simulink model "P41"  (R2015b)
settings: Solver=VariableStepAuto  StartTime=0.0  StopTime=10  RelTol=1e-3
libraries: fl_lib x19, nesl_utility x3
settings Model: Creator=xmax1946  LastModifiedBy=xmax1946

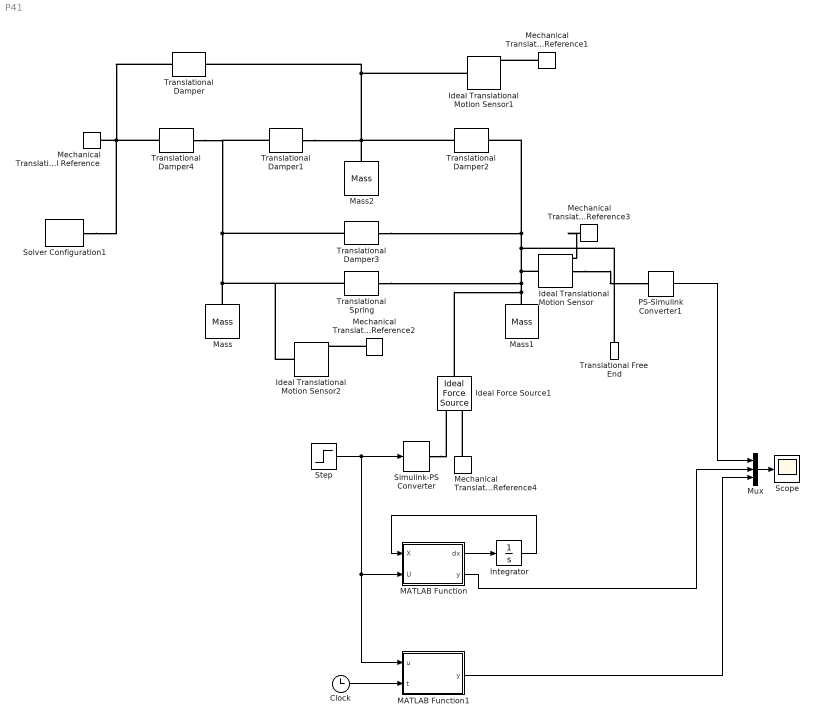
== system P41 ==
  Clock : Clock
  Ideal Force Source1 : fl_lib/Mechanical/Mechanical Sources/Ideal Force Source
  Ideal Translational Motion Sensor : fl_lib/Mechanical/Mechanical Sensors/Ideal Translational Motion Sensor  offset=0 m
  Ideal Translational Motion Sensor1 : fl_lib/Mechanical/Mechanical Sensors/Ideal Translational Motion Sensor  offset=0 m
  Ideal Translational Motion Sensor2 : fl_lib/Mechanical/Mechanical Sensors/Ideal Translational Motion Sensor  offset=0 m
  Integrator : Integrator  InitialCondition=[0;0;0;0;0;0]
  MATLAB Function : MATLAB Function  TreatAsAtomicUnit=on
  MATLAB Function1 : MATLAB Function  TreatAsAtomicUnit=on
  Mass : fl_lib/Mechanical/Translational Elements/Mass  mass=2 kg  v_specify=off  v_priority=None  v=0 m/s  f_specify=off  f_priority=None  f=0 N
  Mass1 : fl_lib/Mechanical/Translational Elements/Mass  mass=1 kg  v_specify=off  v_priority=None  v=0 m/s  f_specify=off  f_priority=None  f=0 N
  Mass2 : fl_lib/Mechanical/Translational Elements/Mass  mass=1 kg  v_specify=off  v_priority=None  v=0 m/s  f_specify=off  f_priority=None  f=0 N
  Mechanical Translational Reference{,1..4} (5 alike) : fl_lib/Mechanical/Translational Elements/Mechanical Translational Reference
  Mux : Mux  Inputs=3
  PS-Simulink Converter1 : nesl_utility/PS-Simulink Converter  PhysicalDomain=network_engine_domain  SubClassName=ps_output  LeftPortType=input  RightPortType=output  PseudoPeriodic=off  Frequencies=[]  Unit=1  AffineConversion=off
  Scope : Scope
  Simulink-PS Converter : nesl_utility/Simulink-PS Converter  PhysicalDomain=network_engine_domain  SubClassName=ps_input  LeftPortType=input  RightPortType=output  PseudoPeriodic=off  Frequencies=[]  NoiseDistribution=none  NoiseParameters=[]  Unit=1  AffineConversion=off  InputFiltering=off  SimscapeFilterOrder=1  InputFilterTimeConstant=0.001  UdotUserProvided=1
  Solver Configuration1 : nesl_utility/Solver Configuration  PhysicalDomain=network_engine_domain  SubClassName=solver  LeftPortType=input  RightPortType=generic  Accelerate=off  Tones=[]  Harmonics=[]  SimulateNoise=off  Profile=off  UseLocalSampling=off  EnableSwitchedLinearOptims=on  FrequencyDomain=off  UseCCode=off  RelTol=0.001  AbsTol=1e-06  MinStep=1e-09  ToWorkspace=off  RevertToSquareIcSolve=off  NumHomotopyIterations=100  PhasorMode=off  PhasorModeNumHarmonics=1  DoDC=off  ResidualTolerance=1e-09  UseLocalSolver=off  LocalSolverChoice=NE_BACKWARD_EULER_ADVANCER  LocalSolverSampleTime=0.001  DoFixedCost=off  MaxNonlinIter=3  MaxModeIter=2  LinearAlgebra=Sparse  DelaysMemoryBudget=1024  AutomaticFiltering=on  FilteringTimeConstant=0.001
  Step : Step  SampleTime=0
  Translational Damper{,1..4} (5 alike) : fl_lib/Mechanical/Translational Elements/Translational Damper  D=1 N/(m/s)  v_specify=off  v_priority=None  v=0 m/s  f_specify=off  f_priority=None  f=0 N
  Translational Free End : fl_lib/Mechanical/Translational Elements/Translational Free End  v_specify=off  v_priority=None  v=0 m/s
  Translational Spring : fl_lib/Mechanical/Translational Elements/Translational Spring  spr_rate=2 N/m  v_specify=off  v_priority=None  v=0 m/s  f_specify=off  f_priority=None  f=0 N  x_specify=off  x_priority=None  x=0 m
  wires:
  Step/1 -> MATLAB Function1/1(u), MATLAB Function/2(U), Simulink-PS Converter/1
  MATLAB Function/1(dx) -> Integrator/1
  MATLAB Function/2(y) -> Mux/2
  PS-Simulink Converter1/1 -> Mux/1
  Mux/1 -> Scope/1
  Integrator/1 -> MATLAB Function/1(X)
  MATLAB Function1/1(y) -> Mux/3
  Clock/1 -> MATLAB Function1/2(t)
  connections:
  Translational Damper4/LConn1 -- Translational Damper/LConn1 -- Mechanical Translational Reference/LConn1 -- Solver Configuration1/RConn1
  Mass/LConn1 -- Translational Damper4/RConn1 -- Translational Damper1/LConn1 -- Translational Damper3/LConn1 -- Ideal Translational Motion Sensor2/LConn1 -- Translational Spring/LConn1
  Mass2/LConn1 -- Translational Damper2/LConn1 -- Translational Damper1/RConn1 -- Ideal Translational Motion Sensor1/LConn1 -- Translational Damper/RConn1
  Mass1/LConn1 -- Ideal Force Source1/LConn1 -- Translational Spring/RConn1 -- Ideal Translational Motion Sensor/LConn1 -- Translational Damper2/RConn1 -- Translational Damper3/RConn1 -- Translational Free End/LConn1
  Mechanical Translational Reference4/LConn1 -- Ideal Force Source1/RConn2
  Simulink-PS Converter/RConn1 -- Ideal Force Source1/RConn1
  Mechanical Translational Reference3/LConn1 -- Ideal Translational Motion Sensor/RConn1
  Mechanical Translational Reference1/LConn1 -- Ideal Translational Motion Sensor1/RConn1
  Mechanical Translational Reference2/LConn1 -- Ideal Translational Motion Sensor2/RConn1
  Ideal Translational Motion Sensor/RConn2 -- PS-Simulink Converter1/LConn1

== matlab function P41/MATLAB Function1 ==
  data: u input; y output; t input
function y = fex(u,t)
if(t<1)
y=0;
else
y=(0.83809356275289271277054931524308*u*exp(-0.47919099197203273069817230426141*t)*(exp(0.47919099197203273069817230426141*t) - 1.0) - 5.8031360760876196553674741324981e-33*u*exp(-0.47919099197203273069817230426141*t)*(exp(3.599210287224430707887196392472*t) - 1.0) + 1.5179259097290730585144913899967*u*exp(-3.599210287224430707887196392472*t)*(exp(3.599210287224430707887196392472*t) - 1.0) - 2.8115447360101444443465915445074e-33*u*exp(-3.599210287224430707887196392472*t)*(exp(0.47919099197203273069817230426141*t) - 1.0) - 4.8586189703032449221709456433168e-34*u*exp(-0.47919099197203273069817230426141*t)*(0.000000000000000000000000000000053134833380184455623079327031296*exp(1.2107993604017682807073156516333*t + 1.2107993604017682807073156516333)*(7860292769360121761917859385977.0*cos(1.1970816347993924595502635158906*t + 1.1970816347993924595502635158906) + 7771239749602461657823637107824.0*sin(1.1970816347993924595502635158906*t + 1.1970816347993924595502635158906)) - 1.80192105665830426991604595998) - 1.3963725449064586540346787566802e-33*u*exp(-3.599210287224430707887196392472*t)*(0.000000000000000000000000000000053134833380184455623079327031296*exp(1.2107993604017682807073156516333*t + 1.2107993604017682807073156516333)*(7860292769360121761917859385977.0*cos(1.1970816347993924595502635158906*t + 1.1970816347993924595502635158906) + 7771239749602461657823637107824.0*sin(1.1970816347993924595502635158906*t + 1.1970816347993924595502635158906)) - 1.80192105665830426991604595998) - 1.3282973985716771521886132191926e-33*u*exp(-0.47919099197203273069817230426141*t)*(0.000000000000000000000000000000053134833380184455623079327031296*exp(1.2107993604017682807073156516333*t + 1.2107993604017682807073156516333)*(7771239749602461657823637107824.0*cos(1.1970816347993924595502635158906*t + 1.1970816347993924595502635158906) - 7860292769360121761917859385977.0*sin(1.1970816347993924595502635158906*t + 1.1970816347993924595502635158906)) + 0.7990334525030318642398392062889) + 1.9122245018643579106623838247516e-36*u*exp(-3.599210287224430707887196392472*t)*(0.000000000000000000000000000000053134833380184455623079327031296*exp(1.2107993604017682807073156516333*t + 1.2107993604017682807073156516333)*(7771239749602461657823637107824.0*cos(1.1970816347993924595502635158906*t + 1.1970816347993924595502635158906) - 7860292769360121761917859385977.0*sin(1.1970816347993924595502635158906*t + 1.1970816347993924595502635158906)) + 0.7990334525030318642398392062889) - 0.000000000000000000000000000000016423149269574731446097433591146*u*exp(-1.2107993604017682807073156516333*t)*cos(1.1970816347993924595502635158906*t)*(exp(3.599210287224430707887196392472*t) - 1.0) - 1.9420308734687061572688296315083e-33*u*exp(-1.2107993604017682807073156516333*t)*cos(1.1970816347993924595502635158906*t)*(exp(0.47919099197203273069817230426141*t) - 1.0) + 4.4430840054719936649837553184706e-33*u*exp(-1.2107993604017682807073156516333*t)*sin(1.1970816347993924595502635158906*t)*(exp(3.599210287224430707887196392472*t) - 1.0) + 2.2527133325166117381451364565456e-33*u*exp(-1.2107993604017682807073156516333*t)*sin(1.1970816347993924595502635158906*t)*(exp(0.47919099197203273069817230426141*t) - 1.0) + 0.60189463237136129398627627176676*u*exp(-1.2107993604017682807073156516333*t)*cos(1.1970816347993924595502635158906*t)*(0.000000000000000000000000000000053134833380184455623079327031296*exp(1.2107993604017682807073156516333*t + 1.2107993604017682807073156516333)*(7860292769360121761917859385977.0*cos(1.1970816347993924595502635158906*t + 1.1970816347993924595502635158906) + 7771239749602461657823637107824.0*sin(1.1970816347993924595502635158906*t + 1.1970816347993924595502635158906)) - 1.80192105665830426991604595998) - 0.51319614056397097658207226137634*u*exp(-1.2107993604017682807073156516333*t)*sin(1.1970816347993924595502635158906*t)*(0.000000000000000000000000000000053134833380184455623079327031296*exp(1.2107993604017682807073156516333*t + 1.2107993604017682807073156516333)*(7860292769360121761917859385977.0*cos(1.1970816347993924595502635158906*t + 1.1970816347993924595502635158906) + 7771239749602461657823637107824.0*sin(1.1970816347993924595502635158906*t + 1.1970816347993924595502635158906)) - 1.80192105665830426991604595998) - 0.51319614056397097658207226137634*u*exp(-1.2107993604017682807073156516333*t)*cos(1.1970816347993924595502635158906*t)*(0.000000000000000000000000000000053134833380184455623079327031296*exp(1.2107993604017682807073156516333*t + 1.2107993604017682807073156516333)*(7771239749602461657823637107824.0*cos(1.1970816347993924595502635158906*t + 1.1970816347993924595502635158906) - 7860292769360121761917859385977.0*sin(1.1970816347993924595502635158906*t + 1.1970816347993924595502635158906)) + 0.7990334525030318642398392062889) - 0.60189463237136129398627627176676*u*exp(-1.2107993604017682807073156516333*t)*sin(1.1970816347993924595502635158906*t)*(0.000000000000000000000000000000053134833380184455623079327031296*exp(1.2107993604017682807073156516333*t + 1.2107993604017682807073156516333)*(7771239749602461657823637107824.0*cos(1.1970816347993924595502635158906*t + 1.1970816347993924595502635158906) - 7860292769360121761917859385977.0*sin(1.1970816347993924595502635158906*t + 1.1970816347993924595502635158906)) + 0.7990334525030318642398392062889) - 3.2506469684475916723867032207957);
end

== matlab function P41/MATLAB Function ==
  data: dx output; X input; y output; U input
function [dx,y] = fss(X,U)
m1=2;
m2=1;
m3=1;
v1=1;
v2=1;
v3=1;
v4=1;
v5=1;
k=2;
A=[0,1,0,0,0,0;
  -k/m1,(-v2-v4-v1)/m1,k/m1,v2/m1,0,v4/m1
  0,0,0,1,0,0 
  k/m2,v2/m2,-k/m2,(-v2-v5)/m2,0,v5/m2
  0,0,0,0,0,1
  0,v4/m3,0,v5/m3,0,(-v4-v3-v5)/m3
    ];
B=[0;0;0;1/m2;0;0];
C=[0,0,0,1,0,0];
u=U;
dx=A*X+B*u;
y=C*X;
